simulink model "Parallel_Ideal_Series_Controllers"  (R2024b)
settings: Solver=VariableStepAuto  StartTime=0.0  StopTime=20  RelTol=1e-3
libraries: simulink x1
settings Model: Creator=LEGION  LastModifiedBy=LEGION

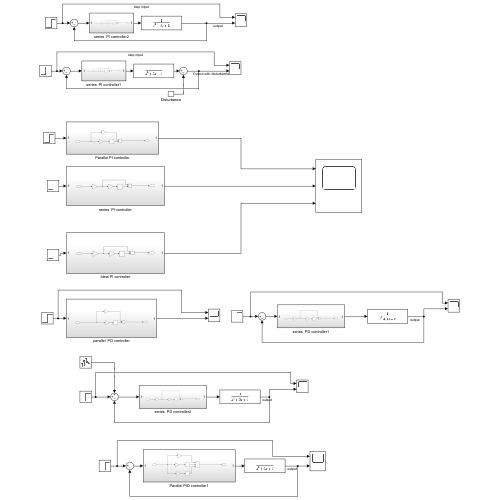
[thumbnail: Simulink's stored preview of the top-level diagram]
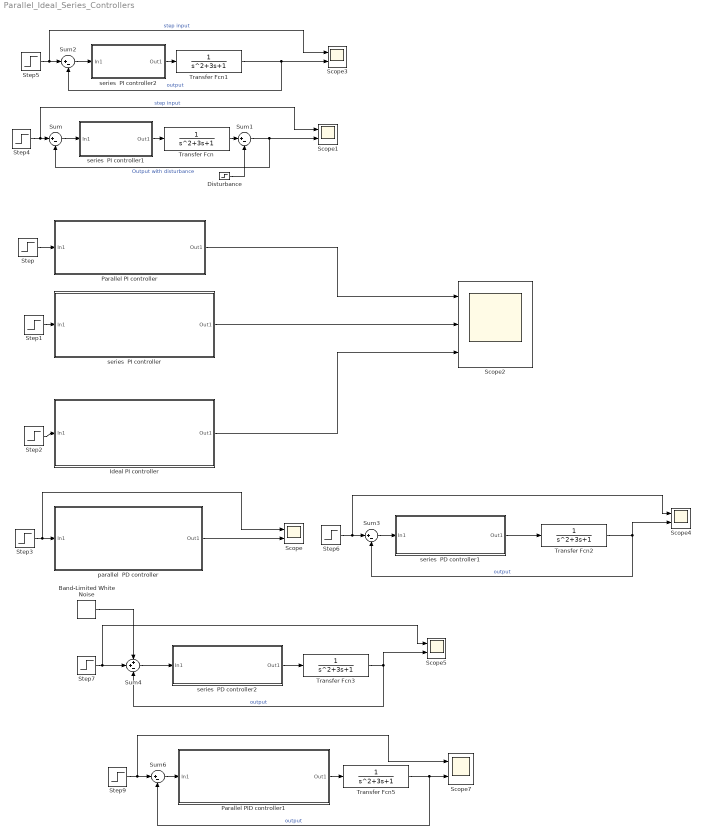
== system Parallel_Ideal_Series_Controllers ==
  Band-Limited White Noise : simulink/Sources/Band-Limited White Noise  Cov=[0.1]  Ts=0.1  seed=[23341]
  Disturbance : Step  Time=5  After=.3  SampleTime=0
  Ideal PI controller : Subsystem
  Parallel PI controller : Subsystem
  Parallel PID controller1 : Subsystem
  Scope{,1,3..5,7} (6 alike) : Scope  NumInputPorts=2
  Scope2 : Scope  NumInputPorts=3
  Step{,1..7,9} (9 alike) : Step  SampleTime=0
  Sum{,1..3,6} (5 alike) : Sum  Inputs=|+-
  Sum4 : Sum  Inputs=++-
  Transfer Fcn{,1..3,5} (5 alike) : TransferFcn  Denominator=[1 3 1]
  parallel  PD controller : Subsystem
  series  PD controller1 : Subsystem
  series  PD controller2 : Subsystem
  series  PI controller : Subsystem
  series  PI controller1 : Subsystem
  series  PI controller2 : Subsystem
  wires:
  series  PI controller/1(Out1) -> Scope2/2
  Parallel PI controller/1(Out1) -> Scope2/1
  Ideal PI controller/1(Out1) -> Scope2/3
  Step/1 -> Parallel PI controller/1(In1)
  Step1/1 -> series  PI controller/1(In1)
  Step2/1 -> Ideal PI controller/1(In1)
  Step3/1 -> Scope/1, parallel  PD controller/1(In1)
  parallel  PD controller/1(Out1) -> Scope/2
  Sum/1 -> series  PI controller1/1(In1)
  series  PI controller1/1(Out1) -> Transfer Fcn/1
  Transfer Fcn/1 -> Sum1/1
  Disturbance/1 -> Sum1/2
  Sum1/1 -> Sum/2, Scope1/2  "Output with disturbance"
  Step4/1 -> Sum/1, Scope1/1  "step input"
  Transfer Fcn1/1 -> Sum2/2, Scope3/2  "output"
  Step5/1 -> Scope3/1, Sum2/1  "step input"
  Sum2/1 -> series  PI controller2/1(In1)
  series  PD controller1/1(Out1) -> Transfer Fcn2/1
  Step6/1 -> Scope4/1, Sum3/1
  series  PI controller2/1(Out1) -> Transfer Fcn1/1
  Transfer Fcn2/1 -> Sum3/2, Scope4/2  "output"
  Sum3/1 -> series  PD controller1/1(In1)
  Step7/1 -> Scope5/1, Sum4/2
  series  PD controller2/1(Out1) -> Transfer Fcn3/1
  Transfer Fcn3/1 -> Scope5/2, Sum4/3  "output"
  Sum4/1 -> series  PD controller2/1(In1)
  Band-Limited White Noise/1 -> Sum4/1
  Step9/1 -> Sum6/1, Scope7/1
  Parallel PID controller1/1(Out1) -> Transfer Fcn5/1
  Transfer Fcn5/1 -> Sum6/2, Scope7/2  "output"
  Sum6/1 -> Parallel PID controller1/1(In1)

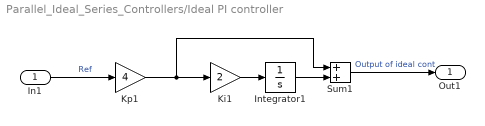
== system Parallel_Ideal_Series_Controllers/Ideal PI controller ==
  In1 : Inport
  Integrator1 : Integrator
  Ki1 : Gain  Gain=2
  Kp1 : Gain  Gain=4
  Sum1 : Sum  Inputs=+|+
  Out1 : Outport
  wires:
  Integrator1/1 -> Sum1/2
  Kp1/1 -> Sum1/1, Ki1/1
  Ki1/1 -> Integrator1/1
  Sum1/1 -> Out1/1  "Output of ideal cont"
  In1/1 -> Kp1/1  "Ref"

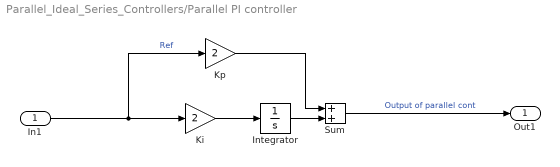
== system Parallel_Ideal_Series_Controllers/Parallel PI controller ==
  In1 : Inport
  Integrator : Integrator
  Ki : Gain  Gain=2
  Kp : Gain  Gain=2
  Sum : Sum  Inputs=+|+
  Out1 : Outport
  wires:
  Integrator/1 -> Sum/2
  In1/1 -> Ki/1, Kp/1  "Ref"
  Ki/1 -> Integrator/1
  Kp/1 -> Sum/1
  Sum/1 -> Out1/1  "Output of parallel cont"

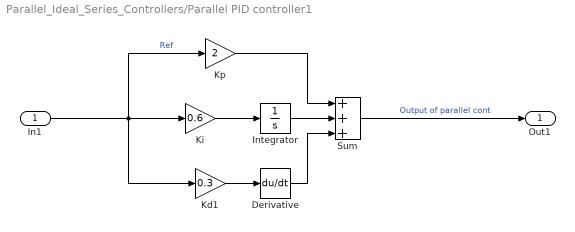
== system Parallel_Ideal_Series_Controllers/Parallel PID controller1 ==
  In1 : Inport
  Derivative : Derivative
  Integrator : Integrator
  Kd1 : Gain  Gain=0.3
  Ki : Gain  Gain=0.6
  Kp : Gain  Gain=2
  Sum : Sum  Inputs=+++
  Out1 : Outport
  wires:
  Integrator/1 -> Sum/2
  In1/1 -> Kd1/1, Ki/1, Kp/1  "Ref"
  Ki/1 -> Integrator/1
  Kp/1 -> Sum/1
  Sum/1 -> Out1/1  "Output of parallel cont"
  Kd1/1 -> Derivative/1
  Derivative/1 -> Sum/3

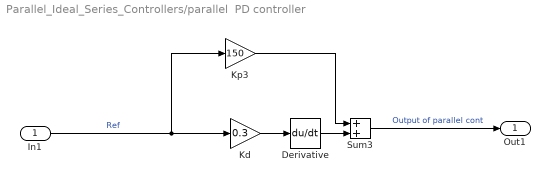
== system Parallel_Ideal_Series_Controllers/parallel  PD controller ==
  In1 : Inport
  Derivative : Derivative
  Kd : Gain  Gain=0.3
  Kp3 : Gain  Gain=150
  Sum3 : Sum  Inputs=+|+
  Out1 : Outport
  wires:
  Sum3/1 -> Out1/1  "Output of parallel cont"
  In1/1 -> Kp3/1, Kd/1  "Ref"
  Kp3/1 -> Sum3/1
  Derivative/1 -> Sum3/2
  Kd/1 -> Derivative/1

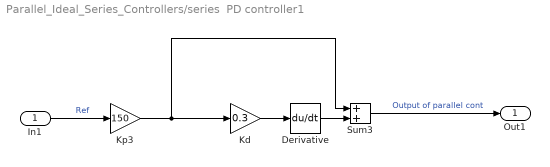
== system Parallel_Ideal_Series_Controllers/series  PD controller1 ==
  In1 : Inport
  Derivative : Derivative
  Kd : Gain  Gain=0.3
  Kp3 : Gain  Gain=150
  Sum3 : Sum  Inputs=+|+
  Out1 : Outport
  wires:
  Sum3/1 -> Out1/1  "Output of parallel cont"
  In1/1 -> Kp3/1  "Ref"
  Derivative/1 -> Sum3/2
  Kd/1 -> Derivative/1
  Kp3/1 -> Sum3/1, Kd/1

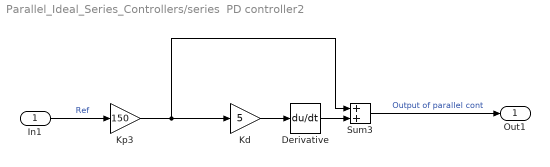
== system Parallel_Ideal_Series_Controllers/series  PD controller2 ==
  In1 : Inport
  Derivative : Derivative
  Kd : Gain  Gain=5
  Kp3 : Gain  Gain=150
  Sum3 : Sum  Inputs=+|+
  Out1 : Outport
  wires:
  Sum3/1 -> Out1/1  "Output of parallel cont"
  In1/1 -> Kp3/1  "Ref"
  Derivative/1 -> Sum3/2
  Kd/1 -> Derivative/1
  Kp3/1 -> Sum3/1, Kd/1

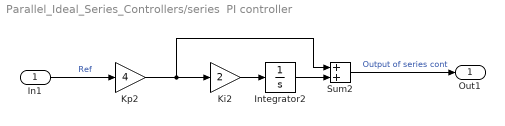
== system Parallel_Ideal_Series_Controllers/series  PI controller ==
  In1 : Inport
  Integrator2 : Integrator
  Ki2 : Gain  Gain=2
  Kp2 : Gain  Gain=4
  Sum2 : Sum  Inputs=+|+
  Out1 : Outport
  wires:
  Ki2/1 -> Integrator2/1
  Kp2/1 -> Sum2/1, Ki2/1
  In1/1 -> Kp2/1  "Ref"
  Integrator2/1 -> Sum2/2
  Sum2/1 -> Out1/1  "Output of series cont"

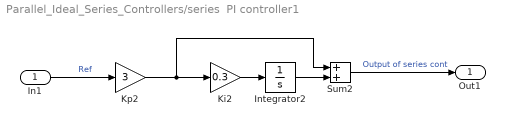
== system Parallel_Ideal_Series_Controllers/series  PI controller1 ==
  In1 : Inport
  Integrator2 : Integrator
  Ki2 : Gain  Gain=0.3
  Kp2 : Gain  Gain=3
  Sum2 : Sum  Inputs=+|+
  Out1 : Outport
  wires:
  Ki2/1 -> Integrator2/1
  Kp2/1 -> Sum2/1, Ki2/1
  In1/1 -> Kp2/1  "Ref"
  Integrator2/1 -> Sum2/2
  Sum2/1 -> Out1/1  "Output of series cont"

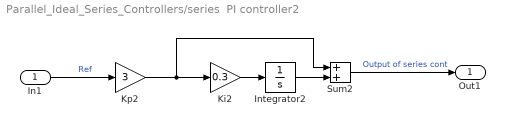
== system Parallel_Ideal_Series_Controllers/series  PI controller2 ==
  In1 : Inport
  Integrator2 : Integrator
  Ki2 : Gain  Gain=0.3
  Kp2 : Gain  Gain=3
  Sum2 : Sum  Inputs=+|+
  Out1 : Outport
  wires:
  Ki2/1 -> Integrator2/1
  Kp2/1 -> Sum2/1, Ki2/1
  In1/1 -> Kp2/1  "Ref"
  Integrator2/1 -> Sum2/2
  Sum2/1 -> Out1/1  "Output of series cont"
